simulink model "part2_2"  (R2021b)
settings: Solver=VariableStepAuto  StartTime=0.0  StopTime=10.0  RelTol=1e-3
settings Model: Creator=setarehdehghanfard  LastModifiedBy=setarehdehghanfard

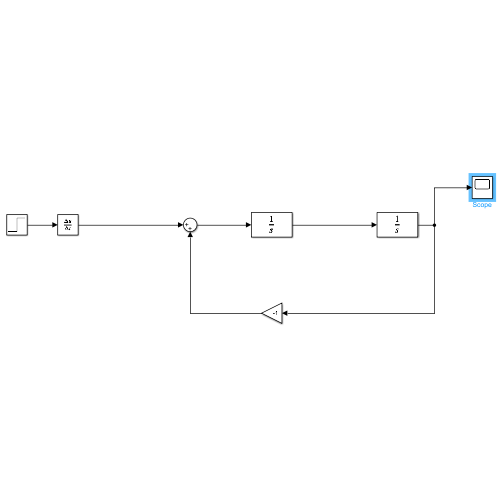
[thumbnail: Simulink's stored preview of the top-level diagram]
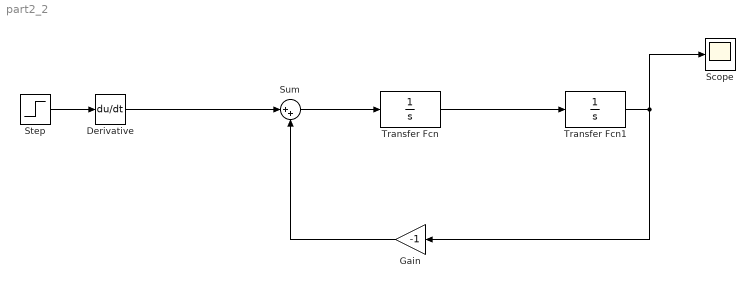
== system part2_2 ==
  Derivative : Derivative
  Gain : Gain  Gain=-1
  Scope : Scope
  Step : Step  Time=0.001  SampleTime=0
  Sum : Sum  Inputs=|++
  Transfer Fcn : TransferFcn  Denominator=[1 0]
  Transfer Fcn1 : TransferFcn  Denominator=[1 0]
  wires:
  Gain/1 -> Sum/2
  Sum/1 -> Transfer Fcn/1
  Derivative/1 -> Sum/1
  Transfer Fcn/1 -> Transfer Fcn1/1
  Step/1 -> Derivative/1
  Transfer Fcn1/1 -> Scope/1, Gain/1
